simulink model "BERvsSNRperbit"  (R2024b)
settings: Solver=VariableStepDiscrete  StartTime=0.0  StopTime=2  MaxStep=1e-3  RelTol=1e-3
libraries: commdigbbndam3 x2, commchan3 x1, simulink x1, commsink2 x1, commrandsrc3 x1
settings Model: Creator=yassi  LastModifiedBy=yassi
settings SolverCC: AlgebraicLoopSolver=TrustRegion
settings DataIOCC: LimitDataPoints=on  SaveOutput=off  SaveTime=off
settings OptimizationCC: BooleanDataType=off  DefaultParameterBehavior=Inlined  LocalBlockOutputs=off  LifeSpan=inf
settings DebuggingCC: AlgebraicLoopMsg=error  SingleTaskRateTransMsg=error  UnconnectedInputMsg=warning  UnconnectedOutputMsg=warning  UnconnectedLineMsg=warning  AllowSymbolicDim=off  SFUnexpectedBacktrackingDiag=warning  SFNoUnconditionalDefaultTransitionDiag=warning  SFExecutionAtInitializationDiag=none  ArithmeticOperatorsInVariantConditions=warning
settings ModelReferenceCC: EnableRefExpFcnMdlSchedulingChecks=on
settings SFSimCC: SimUseLocalCustomCode=off  CustomCodeUndefinedFunction=UseInterfaceOnly
settings RTWCC: RTWUseLocalCustomCode=off  GPUComputeCapability=3.5
settings CodeAppCC: StateflowObjectComments=on
settings GRTTargetCC: TargetLangStandard=C89/C90 (ANSI)
settings ConfigComp: CovMetricSettings=dw  CovSaveCumulativeToWorkspaceVar=on  CovSaveSingleToWorkspaceVar=on  CovExternalEMLEnable=off  CovSFcnEnable=off

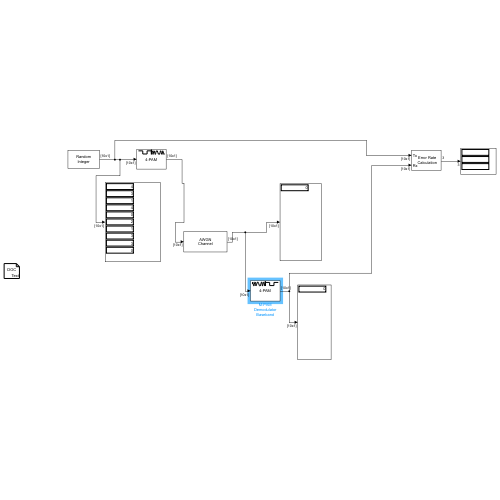
[thumbnail: Simulink's stored preview of the top-level diagram]
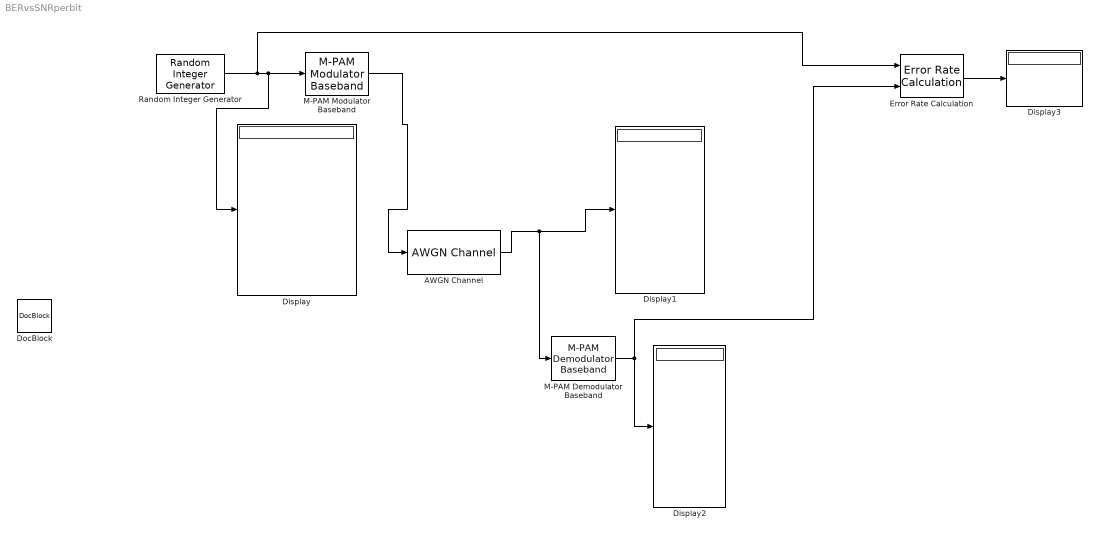
== system BERvsSNRperbit ==
  AWGN Channel : commchan3/AWGN Channel  LegacyMode=off  NoiseMethod="Signal to noise ratio  (Eb/No)"  noiseMode="Signal to noise ratio  (SNR)"  EbNo=10  EsNo=10  SNR=10  BitsPerSymbol=1  SignalPower=1  SamplesPerSymbol=1  SymbolPeriod=1  VarianceSource=Parameter  Variance=1  RandomStream=Global stream  Seed=67  SimulateUsing=Code generation
  Display{,1..3} (4 alike) : Display
  DocBlock : simulink/Model-Wide Utilities/DocBlock  DocumentType=Text
      content=|
      | te3raf te3melha for an analog signal? random int stuff looks too ez
  Error Rate Calculation : commsink2/Error Rate Calculation  N=0  st_delay=0  cp_mode=Entire frame  subframe=[]  PMode=Port  WsName=ErrorVec  RsMode2=off  stop=off  numErr=100  maxBits=1e6
      settings: LibrarySourceBlock=|
      | commhdlsink/Error Rate
      | Calculation
  M-PAM Demodulator Baseband : commdigbbndam3/M-PAM Demodulator Baseband  M=4  OutType=Integer  Dec=Gray  PowType=Min. distance between symbols  MinDist=2  AvgPow=1  PeakPow=1  outDtype1=Inherit via internal rule  outDtype2=Inherit via internal rule  denormFactorWordLen=16  denormFactorDataTypeStr=Inherit: Same word length as input  denormFactorLastDataTypeStr=Inherit: Same word length as input  prodOutWordLen=16  prodOutRoundingMode=Floor  prodOutOverflowMode=Wrap  prodOutOvFlMode=off  prodOutOvFlModeLastStrValue=off  sumWordLen=16
  M-PAM Modulator Baseband : commdigbbndam3/M-PAM Modulator Baseband  M=4  InType=Integer  Enc=Gray  PowType=Min. distance between symbols  MinDist=2  AvgPow=1  PeakPow=1  outDtype=double  outWordLen=16  outUDDataType=sfix(16)  outFracLenMode=Best precision  outFracLen=15  outDataTypeStr=double  outLastDataTypeStr=double
  Random Integer Generator : commrandsrc3/Random Integer Generator  SetSize=4  SeedSource=Auto  Seed=0  SampleTime=10  SamplesPerFrame=10  OutputDataType=double  SimulateUsing=Interpreted execution
  wires:
  M-PAM Modulator Baseband/1 -> AWGN Channel/1
  Random Integer Generator/1 -> Error Rate Calculation/1, Display/1, M-PAM Modulator Baseband/1
  AWGN Channel/1 -> M-PAM Demodulator Baseband/1, Display1/1
  M-PAM Demodulator Baseband/1 -> Display2/1, Error Rate Calculation/2
  Error Rate Calculation/1 -> Display3/1
